simulink model "jun_in_state"  (R2018a)
settings: Solver=VariableStepAuto  StartTime=0.0  StopTime=0.1  RelTol=1e-3
settings Model: Creator=BEAR  LastModifiedBy=BEAR

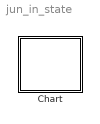
== system jun_in_state ==
  Chart : Stateflow chart  TreatAsAtomicUnit=on

== stateflow chart jun_in_state/Chart ==
  settings: updateMethod=DISCRETE  sampleTime=0.1
  state A
    en:f("enA")
    du:f("duA")
    ex:f("exA")
    state A1
      en:f("enA1")
      ex:f("exA1")
    (default) -> A1
  state C
    en:f("enC")
    du:f("duC")
    ex:f("exC")
    state C2
      en:f("enC2")
      du:f("duC2")
      ex:f("exC2")
  state B
    en:f("enB")
    du:f("duB")
    ex:f("exB")
  (default) -> A
  A1 -> (junction 13) : {f("c1")}/{f("t1")}
  (junction 13) -> C2 : {f("c2")}/{f("t2")}
  data: s function_input
  function f(s):
    | function f(s)
    |     fprintf(s+"\n");
